simulink model "problem2"  (R2023a)
settings: Solver=VariableStepAuto  StartTime=0.0  StopTime=100.0  RelTol=1e-3
undefined symbols (not defined in the file): Cnb0, pitch, roll, x0, yaw
libraries: matrix_library x1
settings Model: Creator=prafulsigdel  LastModifiedBy=prafulsigdel

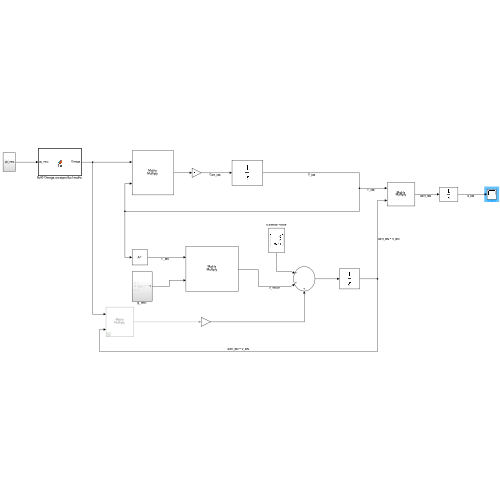
[thumbnail: Simulink's stored preview of the top-level diagram]
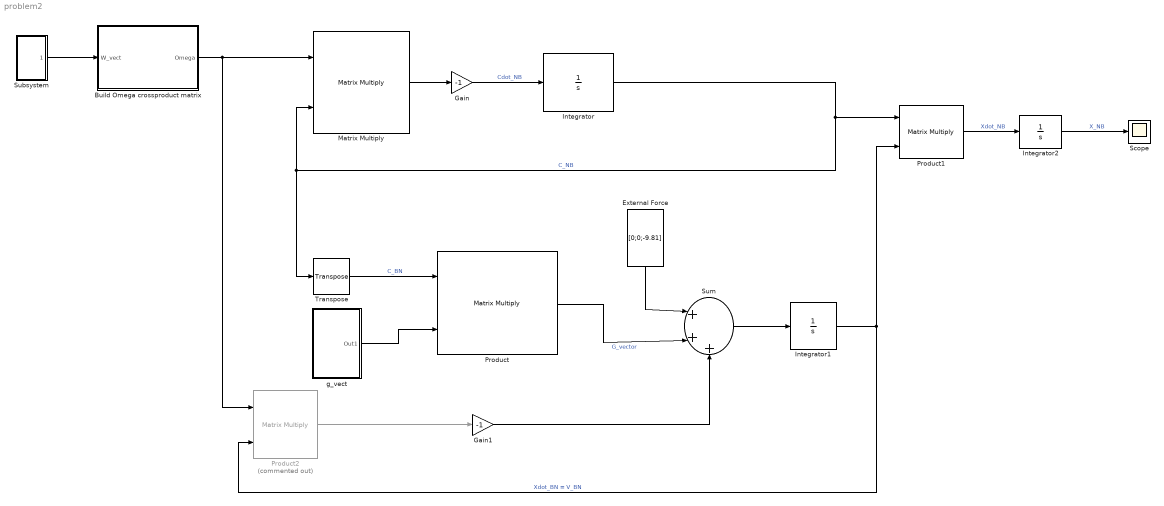
== system problem2 ==
  "Build Omega crossproduct matrix " : MATLAB Function  TreatAsAtomicUnit=on
  External Force : Constant  Value=[0;0;-9.81]  VectorParams1D=off
  Gain : Gain  Gain=-1
  Gain1 : Gain  Gain=-1
  Integrator : Integrator  InitialCondition=Cnb0
  Integrator1 : Integrator  InitialCondition=[150;0;0]
  Integrator2 : Integrator  InitialCondition=x0
  Matrix Multiply : Product  Multiplication=Matrix(*)
  Product : Product  Multiplication=Matrix(*)
  Product1 : Product  Multiplication=Matrix(*)
  Product2 : Product  Commented=on  Multiplication=Matrix(*)
  Scope : Scope
  Subsystem : Subsystem
  Sum : Sum  Inputs=|+++
  Transpose : matrix_library/Transpose
  g_vect : Subsystem
  wires:
  Matrix Multiply/1 -> Gain/1
  "Build Omega crossproduct matrix "/1(Omega) -> Matrix Multiply/1, Product2/1
  Integrator/1 -> Product1/1, Transpose/1, Matrix Multiply/2  "C_NB"
  Subsystem/1(W_vect) -> "Build Omega crossproduct matrix "/1(W_vect)
  Gain/1 -> Integrator/1  "Cdot_NB"
  g_vect/1(Out1) -> Product/2
  Transpose/1 -> Product/1  "C_BN"
  Product/1 -> Sum/2  "G_vector"
  External Force/1 -> Sum/1
  Sum/1 -> Integrator1/1
  Integrator1/1 -> Product2/2, Product1/2  "Xdot_BN = V_BN"
  Product1/1 -> Integrator2/1  "Xdot_NB"
  Integrator2/1 -> Scope/1  "X_NB"
  Product2/1 -> Gain1/1
  Gain1/1 -> Sum/3

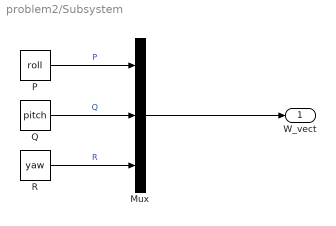
== system problem2/Subsystem ==
  Mux : Mux  Inputs=3
  P : Constant  Value=roll  VectorParams1D=off
  Q : Constant  Value=pitch
  R : Constant  Value=yaw
  W_vect : Outport
  wires:
  P/1 -> Mux/1  "P"
  R/1 -> Mux/3  "R"
  Q/1 -> Mux/2  "Q"
  Mux/1 -> W_vect/1

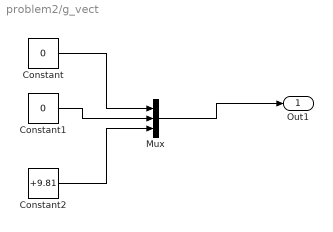
== system problem2/g_vect ==
  Constant : Constant  Value=0
  Constant1 : Constant  Value=0
  Constant2 : Constant  Value=+9.81
  Mux : Mux  Inputs=3
  Out1 : Outport
  wires:
  Constant2/1 -> Mux/3
  Constant/1 -> Mux/1
  Constant1/1 -> Mux/2
  Mux/1 -> Out1/1

== matlab function problem2/Build Omega crossproduct matrix  ==
  data: W_vect input; Omega output
function Omega = fcn(W_vect)

p = W_vect(1);
q = W_vect(2);
r = W_vect(3);


Omega = [0 -r q;
    r 0 -p;
    -q p 0];
